simulink model "closed_loop_LQG"  (R2020a)
settings: Solver=VariableStepAuto  StartTime=0.0  StopTime=50  RelTol=1e-3
undefined symbols (not defined in the file): A1, B1, C1, ctrl_z, inner_h, K, L, omega_max_lim, omega_min_lim, sample_time
libraries: simulink x1
settings Model: Creator=martinhe  LastModifiedBy=martinhe

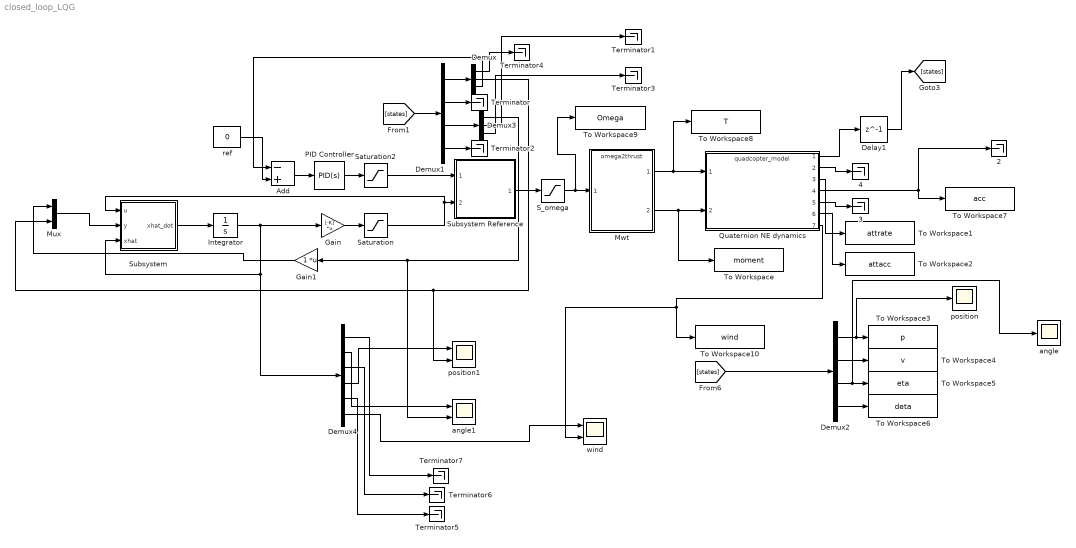
== system closed_loop_LQG ==
  "   2" : Terminator
  "   3" : Terminator
  "   4" : Terminator
  Add : Sum  Inputs=-+
  Delay1 : Delay  DelayLength=1  SampleTime=inner_h
  Demux : Demux  Outputs=3
  Demux1 : Demux  Outputs=[3,3,3,3]
  Demux2 : Demux  Outputs=[3,3,3,3]
  Demux3 : Demux  Outputs=3
  Demux4 : Demux  Outputs=[1 1 1 1 1 1]
  Gain : Gain  Gain=[-K]  Multiplication=Matrix(K*u)
  Gain1 : Gain  Multiplication=Matrix(K*u)
  Integrator : Integrator  InitialCondition=zeros(6,1)
  Mux : Mux  Inputs=2
  Mwt : ModelReference  ModelNameDialog=omega2thrust.mdl  SimulationMode=Normal  ModelReferenceVersion=1.5
  PID Controller : simulink/Continuous/PID Controller  Controller=PID  Form=Parallel  TimeDomain=Continuous-time  UseExternalTs=off  SampleTime=-1  IntegratorMethod=Forward Euler  FilterMethod=Forward Euler  ControllerParametersSource=internal  P=ctrl_z.Kp  I=ctrl_z.Ki  D=ctrl_z.Kd  UseFilter=on  N=100  TunerSelectOption=Transfer Function Based (PID Tuner App)  InitialConditionSource=internal  InitialConditionForIntegrator=0  InitialConditionForFilter=0  DifferentiatorICPrevScaledInput=0  ExternalReset=none  TrackingMode=off  Kt=1  LimitOutput=off  UpperSaturationLimit=inf  LowerSaturationLimit=-inf  LinearizeAsGain=on  AntiWindupMode=none  Kb=1  POutMin=[]  POutMax=[]  IOutMin=[]  IOutMax=[]  DOutMin=[]  DOutMax=[]  NOutMin=[]  NOutMax=[]  SumOutMin=[]  SumOutMax=[]  SaturationOutMin=[]  SaturationOutMax=[]  PParamMin=[]  PParamMax=[]  IParamMin=[]  IParamMax=[]  DParamMin=[]  DParamMax=[]  NParamMin=[]  NParamMax=[]  KbParamMin=[]  KbParamMax=[]  KtParamMin=[]  KtParamMax=[]  KbOutMin=[]  KbOutMax=[]  KtOutMin=[]  KtOutMax=[]  IntegratorOutMin=[]  IntegratorOutMax=[]  FilterOutMin=[]  FilterOutMax=[]  SumI1OutMin=[]  SumI1OutMax=[]  SumI2OutMin=[]  SumI2OutMax=[]  SumI3OutMin=[]  SumI3OutMax=[]  SumI4OutMin=[]  SumI4OutMax=[]  SumDOutMin=[]  SumDOutMax=[]  DifferentiatorOutMin=[]  DifferentiatorOutMax=[]  FilterDiffOutCoefMin=[]  FilterDiffOutCoefMax=[]  ReciprocalOutMin=[]  ReciprocalOutMax=[]  SumDenOutMin=[]  SumDenOutMax=[]  SumNumOutMin=[]  SumNumOutMax=[]  DivideOutMin=[]  DivideOutMax=[]  UdiffTsProdOutMin=[]  UdiffTsProdOutMax=[]  NTsProdOutMin=[]  NTsProdOutMax=[]  UintegralTsProdOutMin=[]  UintegralTsProdOutMax=[]  UngainTsProdOutMin=[]  UngainTsProdOutMax=[]  IntegratorContinuousStateAttributes=''  IntegratorStateMustResolveToSignalObject=off  IntegratorRTWStateStorageClass=Auto  FilterContinuousStateAttributes=''  FilterStateMustResolveToSignalObject=off  FilterRTWStateStorageClass=Auto  ParallelPVariant=InternalParameters  IdealPVariant=Disabled  IVariant=InternalParameters  DVariant=InternalParameters  IntegratorVariant=Continuous  SatVariant=Disabled  AWVariant=Passthrough  PCopyVariant=Disabled  TRVariant=Disabled  FdbkBlocksVariant=Forward  IdealPFdbkVariant=Disabled  SatFdbkVariant=Disabled  DerivativeFilterVariant=ContFilter  NVariant=InternalParameters  NCopyVariant=Disabled  FilterICVariant=InternalICsFilter  IntegratorICVariant=InternalICs  ExternalResetVariant=Disabled  TRSumVariant=Passthrough  SumFdbkVariant=Disabled  SumVariant=Sum_PID  TsampFilterVariant=InternalTs  TsampNgainVariant=Passthrough  TsampIntegralVariant=Passthrough
  Quaternion NE dynamics : ModelReference  ModelNameDialog=quadcopter_model.mdl  SimulationMode=Normal  ModelReferenceVersion=1.340
  S_omega : Saturate  UpperLimit=omega_max_lim  LowerLimit=omega_min_lim
  Saturation : Saturate  UpperLimit=1e-3  LowerLimit=-1e-3
  Saturation2 : Saturate  UpperLimit=inf  LowerLimit=-inf
  Subsystem : Subsystem
  Subsystem Reference : Subsystem  ReferencedSubsystem=thrust2omega
  Terminator{,1..7} (8 alike) : Terminator
  To Workspace : ToWorkspace  VariableName=moment  SaveFormat=Timeseries  SampleTime=sample_time
  To Workspace1 : ToWorkspace  VariableName=attrate  SaveFormat=Timeseries  SampleTime=sample_time
  To Workspace10 : ToWorkspace  VariableName=wind  SaveFormat=Timeseries  SampleTime=sample_time
  To Workspace2 : ToWorkspace  VariableName=attacc  SaveFormat=Timeseries  SampleTime=sample_time
  To Workspace3 : ToWorkspace  VariableName=p  SaveFormat=Timeseries  SampleTime=sample_time
  To Workspace4 : ToWorkspace  VariableName=v  SaveFormat=Timeseries  SampleTime=sample_time
  To Workspace5 : ToWorkspace  VariableName=eta  SaveFormat=Timeseries  SampleTime=sample_time
  To Workspace6 : ToWorkspace  VariableName=deta  SaveFormat=Timeseries  SampleTime=sample_time
  To Workspace7 : ToWorkspace  VariableName=acc  SaveFormat=Timeseries  SampleTime=sample_time
  To Workspace8 : ToWorkspace  VariableName=T  SaveFormat=Timeseries  SampleTime=sample_time
  To Workspace9 : ToWorkspace  VariableName=Omega  SaveFormat=Timeseries  SampleTime=sample_time
  angle : Scope
  angle1 : Scope  NumInputPorts=2
  position : Scope
  position1 : Scope  NumInputPorts=2
  ref : Constant  Value=0
  wind : Scope  NumInputPorts=2
  wires:
  Quaternion NE dynamics/5 -> "   3"/1
  Quaternion NE dynamics/3 -> To Workspace1/1
  Quaternion NE dynamics/6 -> To Workspace2/1
  [states] -> Demux2/1
  Demux2/2 -> To Workspace4/1
  Demux2/3 -> angle/1, To Workspace5/1
  Quaternion NE dynamics/4 -> To Workspace7/1, "   2"/1
  Mwt/1 -> To Workspace8/1, Quaternion NE dynamics/1
  Demux2/1 -> position/1, To Workspace3/1
  S_omega/1 -> To Workspace9/1, Mwt/1
  Quaternion NE dynamics/2 -> "   4"/1
  Mwt/2 -> To Workspace/1, Quaternion NE dynamics/2
  Demux2/4 -> To Workspace6/1
  [states] -> Demux1/1
  Demux1/1 -> Demux/1
  Demux1/2 -> Terminator/1
  Demux1/3 -> Demux3/1
  Demux1/4 -> Terminator2/1
  Subsystem Reference/1 -> S_omega/1
  ref/1 -> Add/2
  Add/1 -> PID Controller/1
  Demux/1 -> Terminator4/1
  Demux/3 -> Add/1
  PID Controller/1 -> Saturation2/1
  Quaternion NE dynamics/7 -> wind/2, To Workspace10/1
  Demux3/1 -> angle1/2, Gain1/1
  Saturation2/1 -> Subsystem Reference/1
  Saturation/1 -> Subsystem/1(u), Subsystem Reference/2
  Gain/1 -> Saturation/1
  Demux4/4 -> position1/1
  Demux4/2 -> angle1/1
  Integrator/1 -> Demux4/1, Subsystem/3(xhat), Gain/1
  Gain1/1 -> Mux/1
  Demux/2 -> position1/2, Mux/2
  Mux/1 -> Subsystem/2(y)
  Subsystem/1(xhat_dot) -> Integrator/1
  Demux4/6 -> wind/1
  Quaternion NE dynamics/1 -> Delay1/1
  Delay1/1 -> [states]
  Demux3/2 -> Terminator1/1
  Demux3/3 -> Terminator3/1
  Demux4/1 -> Terminator7/1
  Demux4/3 -> Terminator6/1
  Demux4/5 -> Terminator5/1

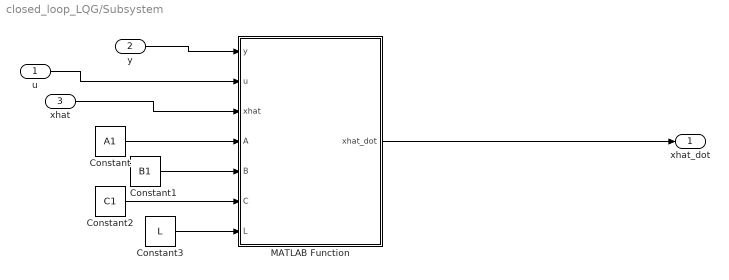
== system closed_loop_LQG/Subsystem ==
  u : Inport
  y : Inport  Port=2
  xhat : Inport  Port=3
  Constant : Constant  Value=A1
  Constant1 : Constant  Value=B1
  Constant2 : Constant  Value=C1
  Constant3 : Constant  Value=L
  MATLAB Function : MATLAB Function  TreatAsAtomicUnit=on
  xhat_dot : Outport
  wires:
  u/1 -> MATLAB Function/2(u)
  y/1 -> MATLAB Function/1(y)
  MATLAB Function/1(xhat_dot) -> xhat_dot/1
  Constant/1 -> MATLAB Function/4(A)
  Constant1/1 -> MATLAB Function/5(B)
  Constant2/1 -> MATLAB Function/6(C)
  Constant3/1 -> MATLAB Function/7(L)
  xhat/1 -> MATLAB Function/3(xhat)

== matlab function closed_loop_LQG/Subsystem/MATLAB Function ==
  data: y input; u input; xhat_dot output; xhat input; A input; B input; C input; L input
function xhat_dot  = kalman(y,u,xhat,A,B,C,L)

xhat_dot = A*xhat+B*u +L*(y-C*xhat) ;
